simulink subsystem "Position_Eq"  (R2022b)
settings: Solver=VariableStepAuto  StartTime=0.0  StopTime=10.0  RelTol=1e-3
settings Model: Creator=MAAM  LastModifiedBy=MAAM

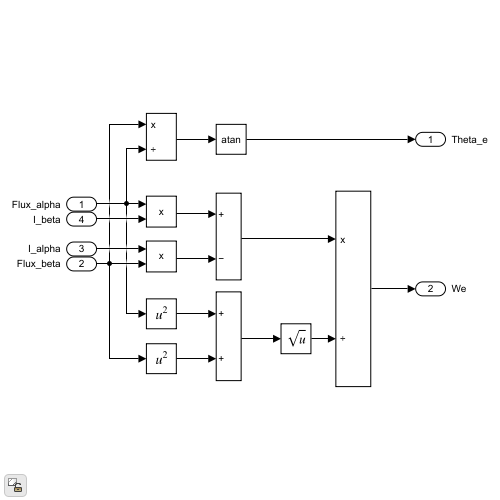
[thumbnail: Simulink's stored preview of the top-level diagram]
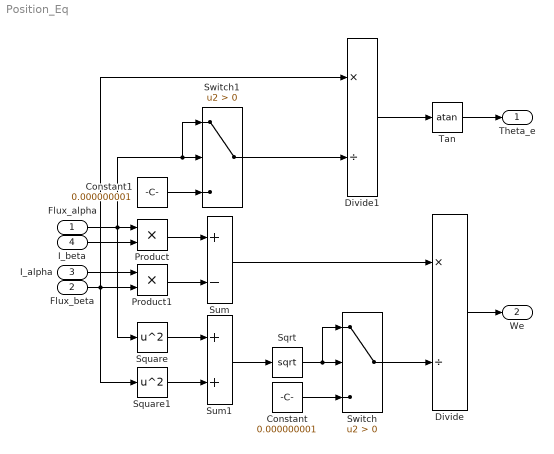
== system Position_Eq ==
  Flux_alpha : Inport
  Flux_beta : Inport  Port=2
  I_alpha : Inport  Port=3
  I_beta : Inport  Port=4
  Constant : Constant  Value=0.000000001
  Constant1 : Constant  Value=0.000000001
  Divide : Product  Inputs=*/
  Divide1 : Product  Inputs=*/
  Product : Product
  Product1 : Product
  Sqrt : Sqrt
  Square : Math  Operator=square
  Square1 : Math  Operator=square
  Sum : Sum  Inputs=+-
  Sum1 : Sum
  Switch : Switch  Criteria=u2 > Threshold  SaturateOnIntegerOverflow=off  InputSameDT=off
  Switch1 : Switch  Criteria=u2 > Threshold  SaturateOnIntegerOverflow=off  InputSameDT=off
  Tan : Trigonometry  Operator=atan
  Theta_e : Outport
  We : Outport  Port=2
  wires:
  I_beta/1 -> Product/2
  Product/1 -> Sum/1
  I_alpha/1 -> Product1/1
  Square1/1 -> Sum1/2
  Sum1/1 -> Sqrt/1
  Product1/1 -> Sum/2
  Divide/1 -> We/1
  Square/1 -> Sum1/1
  Sum/1 -> Divide/1
  Sqrt/1 -> Switch/2, Switch/1
  Switch/1 -> Divide/2
  Constant/1 -> Switch/3
  Tan/1 -> Theta_e/1
  Switch1/1 -> Divide1/2
  Divide1/1 -> Tan/1
  Flux_beta/1 -> Product1/2, Divide1/1, Square1/1
  Constant1/1 -> Switch1/3
  Flux_alpha/1 -> Product/1, Square/1, Switch1/2, Switch1/1
